simulink model "silownik_scheme"  (R2021b)
settings: Solver=VariableStepAuto  StartTime=0.0  StopTime=10.0  RelTol=1e-3
values from neighbouring files (symbols this model uses):
  A_1 = 1688/10^6    (= 0.001688)    [silownik_const.m]
  A_2 = 2*678/10^6    (= 0.001356)    [silownik_const.m]
  K = 1.44 * 10^9    (= 1440000000)    [silownik_const.m]
  m = 4*0.5    (= 2)    [silownik_const.m]
  V_01 = 4*4522/10^9    (= 1.8088e-05)    [silownik_const.m]
  V_02 = 4*102218/10^9    (= 0.000408872)    [silownik_const.m]
settings Model: Creator=szymon_kubuntu  LastModifiedBy=szymon_kubuntu

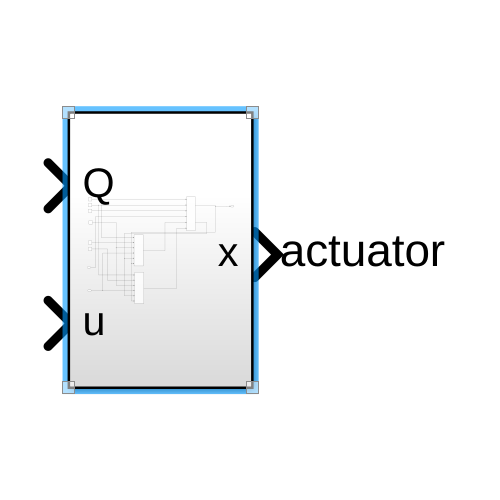
[thumbnail: Simulink's stored preview of the top-level diagram]
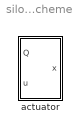
== system silownik_scheme ==
  actuator : Subsystem

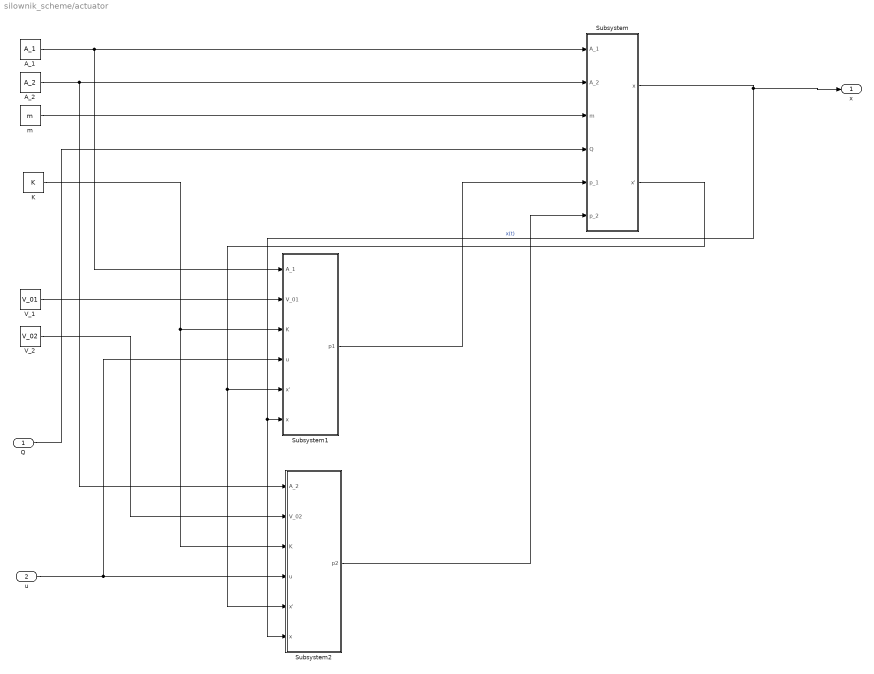
== system silownik_scheme/actuator ==
  Q : Inport
  u : Inport  Port=2
  A_1 : Constant  Value=A_1
  A_2 : Constant  Value=A_2
  K : Constant  Value=K
  Subsystem : Subsystem
  Subsystem1 : Subsystem
  Subsystem2 : Subsystem
  V_1 : Constant  Value=V_01
  V_2 : Constant  Value=V_02
  m : Constant  Value=m
  x : Outport
  wires:
  Subsystem2/1(p2) -> Subsystem/6(p_2)
  V_2/1 -> Subsystem2/2(V_02)
  A_1/1 -> Subsystem1/1(A_1), Subsystem/1(A_1)
  A_2/1 -> Subsystem2/1(A_2), Subsystem/2(A_2)
  Q/1 -> Subsystem/4(Q)
  u/1 -> Subsystem1/4(u), Subsystem2/4(u)
  Subsystem/2(x') -> Subsystem2/5(x'), Subsystem1/5(x')
  K/1 -> Subsystem2/3(K), Subsystem1/3(K)
  Subsystem1/1(p1) -> Subsystem/5(p_1)
  Subsystem/1(x) -> x/1, Subsystem2/6(x), Subsystem1/6(x)  "x(t)"
  V_1/1 -> Subsystem1/2(V_01)
  m/1 -> Subsystem/3(m)

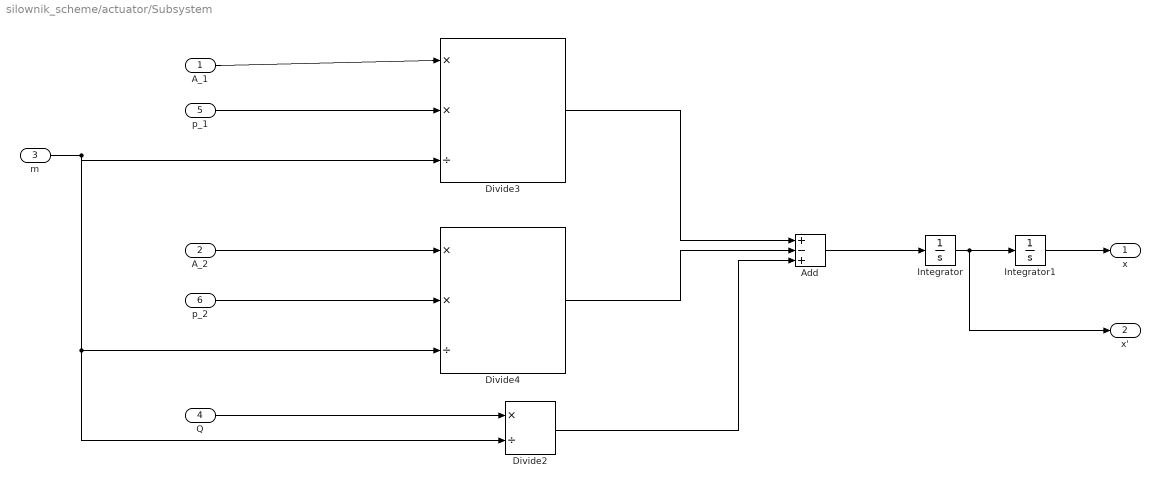
== system silownik_scheme/actuator/Subsystem ==
  A_1 : Inport
  A_2 : Inport  Port=2
  m : Inport  Port=3
  Q : Inport  Port=4
  p_1 : Inport  Port=5
  p_2 : Inport  Port=6
  Add : Sum  Inputs=+-+
  Divide2 : Product  Inputs=*/
  Divide3 : Product  Inputs=**/
  Divide4 : Product  Inputs=**/
  Integrator : Integrator
  Integrator1 : Integrator
  x : Outport
  x' : Outport  Port=2
  wires:
  A_1/1 -> Divide3/1
  p_1/1 -> Divide3/2
  Divide2/1 -> Add/3
  m/1 -> Divide3/3, Divide4/3, Divide2/2
  Q/1 -> Divide2/1
  p_2/1 -> Divide4/2
  A_2/1 -> Divide4/1
  Divide3/1 -> Add/1
  Divide4/1 -> Add/2
  Add/1 -> Integrator/1
  Integrator/1 -> x'/1, Integrator1/1
  Integrator1/1 -> x/1

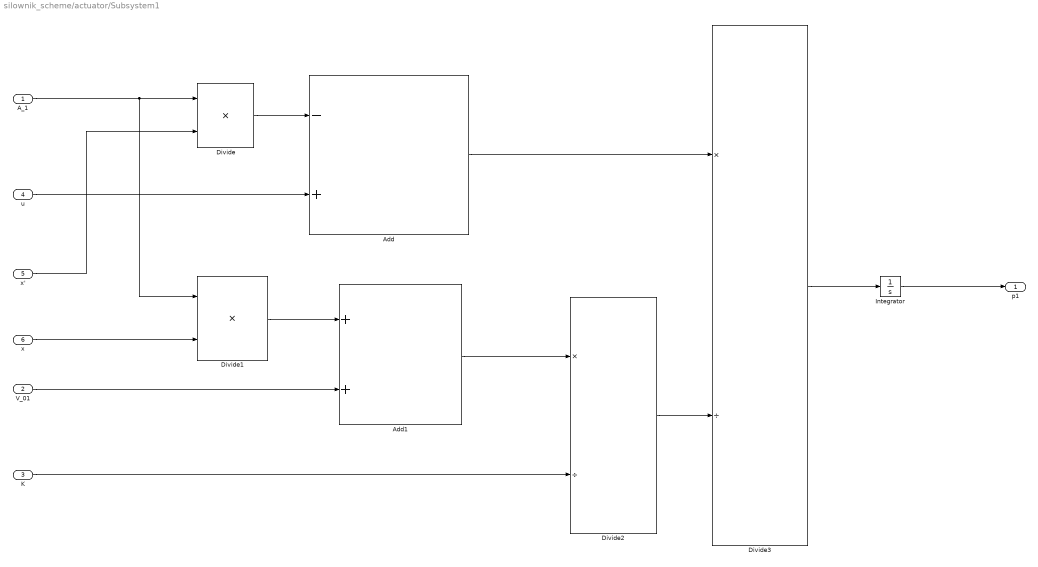
== system silownik_scheme/actuator/Subsystem1 ==
  A_1 : Inport
  V_01 : Inport  Port=2
  K : Inport  Port=3
  u : Inport  Port=4
  x' : Inport  Port=5
  x : Inport  Port=6
  Add : Sum  Inputs=-+
  Add1 : Sum
  Divide : Product  Inputs=**
  Divide1 : Product  Inputs=**
  Divide2 : Product  Inputs=*/
  Divide3 : Product  Inputs=*/
  Integrator : Integrator
  p1 : Outport
  wires:
  A_1/1 -> Divide1/1, Divide/1
  x'/1 -> Divide/2
  Divide/1 -> Add/1
  u/1 -> Add/2
  x/1 -> Divide1/2
  Divide1/1 -> Add1/1
  V_01/1 -> Add1/2
  Add1/1 -> Divide2/1
  K/1 -> Divide2/2
  Add/1 -> Divide3/1
  Divide2/1 -> Divide3/2
  Divide3/1 -> Integrator/1
  Integrator/1 -> p1/1

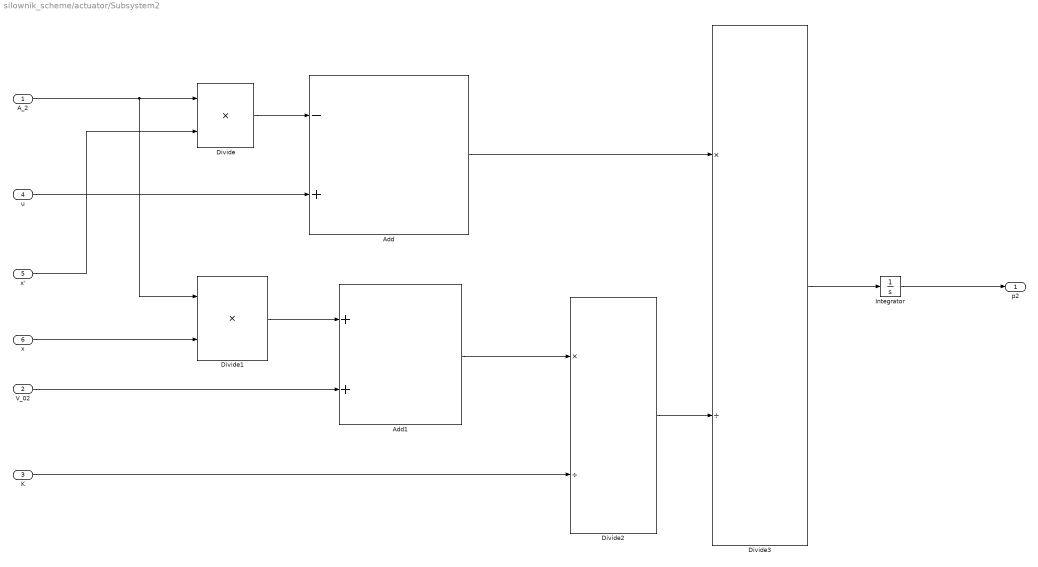
== system silownik_scheme/actuator/Subsystem2 ==
  A_2 : Inport
  V_02 : Inport  Port=2
  K : Inport  Port=3
  u : Inport  Port=4
  x' : Inport  Port=5
  x : Inport  Port=6
  Add : Sum  Inputs=-+
  Add1 : Sum
  Divide : Product  Inputs=**
  Divide1 : Product  Inputs=**
  Divide2 : Product  Inputs=*/
  Divide3 : Product  Inputs=*/
  Integrator : Integrator
  p2 : Outport
  wires:
  Integrator/1 -> p2/1
  Divide3/1 -> Integrator/1
  Divide2/1 -> Divide3/2
  Add/1 -> Divide3/1
  K/1 -> Divide2/2
  Add1/1 -> Divide2/1
  V_02/1 -> Add1/2
  Divide1/1 -> Add1/1
  x/1 -> Divide1/2
  u/1 -> Add/2
  Divide/1 -> Add/1
  x'/1 -> Divide/2
  A_2/1 -> Divide/1, Divide1/1
